simulink library "sm_scissor_lift_lib"  (R2020a)
settings: Solver=ode45  StartTime=0.0  StopTime=10.0  RelTol=1e-3  EnableMultiTasking=on
undefined symbols (not defined in the file): Extr_Data_Ring, Local, SCL_Par, X, Y, Z
libraries: sm_lib x38, $bdroot x37
(part 1 of 2)
Description:
  | Copyright 2014-2020 The MathWorks, Inc.
settings Model: Creator=smiller  LastModifiedBy=Vulca
settings DataIOCC: LimitDataPoints=on  SaveFormat=Array  SignalLoggingSaveFormat=ModelDataLogs  ReturnWorkspaceOutputs=off
settings OptimizationCC: ExpressionDepthLimit=2147483647  LifeSpan=inf
settings DebuggingCC: UnderspecifiedInitializationDetection=Classic  MergeDetectMultiDrivingBlocksExec=none  SolverPrmCheckMsg=warning  FcnCallInpInsideContextMsg=warning  AllowSymbolicDim=off  StateNameClashWarn=warning  PregeneratedLibrarySubsystemCodeDiagnostic=none  SFUnexpectedBacktrackingDiag=warning  SFNoUnconditionalDefaultTransitionDiag=warning  SFExecutionAtInitializationDiag=none  ArithmeticOperatorsInVariantConditions=warning
settings HardwareCC: ProdBitPerPointer=32  ProdBitPerSizeT=32  ProdBitPerPtrDiffT=32  ProdLargestAtomicFloat=None  ProdIntDivRoundTo=Undefined  ProdEndianess=Unspecified  ProdWordSize=32  ProdHWDeviceType=32-bit Generic
settings ModelReferenceCC: PropagateSignalLabelsOutOfModel=off
settings SFSimCC: SimUseLocalCustomCode=off  CustomCodeUndefinedFunction=UseInterfaceOnly
settings RTWCC: RTWUseLocalCustomCode=off
settings CodeAppCC: StateflowObjectComments=on
settings GRTTargetCC: TargetLangStandard=C89/C90 (ANSI)
settings ConfigComp: CovMetricSettings=dw  CovHtmlReporting=on  CovSaveCumulativeToWorkspaceVar=on  CovSaveSingleToWorkspaceVar=on  CovExternalEMLEnable=off  CovSFcnEnable=off

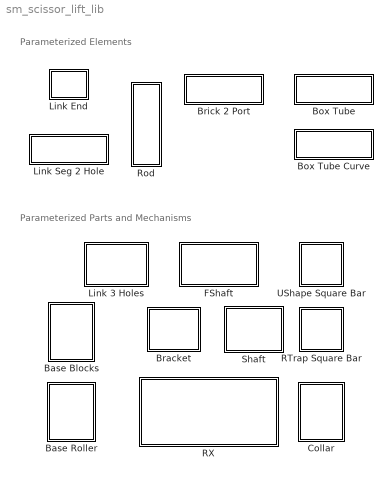
== system sm_scissor_lift_lib ==
  note: Parameterized Elements
  note: Parameterized Parts and Mechanisms
  Base Blocks : Subsystem  mask(Base Blocks){block_length=SCL_Par.Base_Block.Length, block_width=SCL_Par.Base_Block.Width, block_height=SCL_Par.Base_Block.Height, shaft_radius=SCL_Par.Roller.Shaft_Radius, shaft_length=SCL_Par.Roller.Shaft_Length, material_density=SCL_Par.Base_Block.Density, material_color=SCL_Par.Base_Block.Color, material_opacity=SCL_Par.Base_Block.Opacity}
      mask prompts: block_length "Length (cm)"; block_width "Width (cm)"; block_height "Height (cm)"; shaft_radius "Radius (cm)"; shaft_length "Length (cm)"; material_density "Density (kg/m^3)"; material_color "Color [RGB]"; material_opacity "Opacity (0-1)"
      mask help: Parameterized base with two blocks and a shaft.
      mask DialogControl ParameterTabVar0 Prompt: Block
      mask DialogControl ParameterTabVar01 Prompt: Shaft
      mask DialogControl ParameterTabVar012 Prompt: Material
      mask Display: image('Base_Blocks_IMAGE.jpg');
  Base Roller : Subsystem  mask(Base Roller){roller_length=SCL_Par.Roller.Roller_Length, roller_radius=SCL_Par.Roller.Roller_Radius, shaft_length=SCL_Par.Roller.Shaft_Length, shaft_radius=SCL_Par.Roller.Shaft_Radius, material_density=SCL_Par.Roller.Density, material_color=SCL_Par.Roller.Color, material_opacity=SCL_Par.Roller.Opacity}
      mask prompts: roller_length "Length (cm)"; roller_radius "Radius (cm)"; shaft_length "Length (cm)"; shaft_radius "Radius (cm)"; material_density "Density (kg/m^3)"; material_color "Color [RGB]"; material_opacity "Opacity (0-1)"
      mask help: Parameterized roller with two wheels connected by a shaft.
      mask DialogControl ParameterTabVar0 Prompt: Roller
      mask DialogControl ParameterTabVar01 Prompt: Shaft
      mask DialogControl ParameterTabVar012 Prompt: Material
      mask Display: image('Base_Roller_IMAGE.jpg');
  Box Tube : Subsystem  mask(Box Tube){box_ox=0.02, box_ix=0.01, box_oy=0.028, box_iy=0.018, box_len=0.5, box_rho=7000, box_color=[0 0.4 0.6], box_opc=1}
      mask prompts: box_len "Length (m)"; box_rho "Density (kg/m^3)"; box_color "Color [RGB]"; box_opc "Opacity (0-1)"
      mask help: Box tube. Define outer dimensions, inner dimensions, and length. Length defines the distance of the +X frame from the X frame along the x-axis.
      mask init:
      | box_xsec = Extr_Data_Box(box_ox, box_ix, box_oy, box_iy);
      mask DialogControl Control12 Prompt: Plot Profile
      mask DialogControl Control12 Callback:
      | v = get_param(gcb,'MaskWSVariables');
      | getMaskValue = containers.Map({v.Name}',{v.Value}');
      | evalin('base',...
      |     sprintf('Extr_Data_Box(%s,%s,%s,%s,''%s'');',...
      |     num2str(getMaskValue('box_ox')),...
      |     num2str(getMaskValue('box_ix')),...
      |     num2str(getMaskValue('box_oy')),...
      |     num2str(getMaskValue('box_iy')),'plot'));
      mask DialogControl Control3 Prompt: Outer
      mask DialogControl Control4 Prompt: Inner
      mask DialogControl Control5 Prompt: Width (m)
      mask DialogControl Control6 Prompt: Height (m)
      mask Display: image('Box_Tube_IMAGE.png');
  Box Tube Curve : Subsystem  mask(Box Tube with Curve){box_ox=0.02, box_ix=0.01, box_oy=0.028, box_iy=0.018, arc_rad=0.5, arc_angle=-60, popup_arcdir=Y, box_rho=7000, box_color=[0 0.4 0.6], box_opc=1}
      mask prompts: arc_rad "Arc Radius (m)"; arc_angle "Arc Angle (deg)"; popup_arcdir "About"; box_rho "Density (kg/m^3)"; box_color "Color [RGB]"; box_opc "Opacity (0-1)"
      mask help: Box tube. Define outer dimensions, inner dimensions, and length. Length defines the distance of the F frame from the B frame along the z-axis.
      mask init:
      | box_xsec = Extr_Data_Box(box_ox, box_ix, box_oy, box_iy);
      | 
      | % Transform extrusion data based on curve axis and direction
      | if (arc_angle<0)
      |     if(strcmpi(get_param(gcb,'popup_arcdir'),'y'))
      |         box_xsec_d = flipud(box_xsec.*[1 -1]);
      |         Bzrot = -90-arc_angle/2;
      |         Fzrot = -90+arc_angle/2;
      |     elseif(strcmpi(get_param(gcb,'popup_arcdir'),'z'))
      |         box_xsec_d = fliplr(box_xsec).*[1 -1];
      |         Bzrot = 90+arc_angle/2;
      |         Fzrot = -90+arc_angle/2;
      |     end
      | else
      |     if(strcmpi(get_param(gcb,'popup_arcdir'),'y'))
      |         box_xsec_d = flipud(box_xsec.*[-1 1]);
      |     elseif(strcmpi(get_param(gcb,'popup_arcdir'),'z'))
      |         box_xsec_d = -flipud(fliplr(box_xsec));
      |     end
      |     Bzrot = -90+arc_angle/2;
      |     Fzrot = 90+arc_angle/2;
      | end
      | 
      | % Add offset for arc radius
      | box_xsec_d = box_xsec_d + [arc_rad 0];
      | 
      | % Adjust Base and Follower transforms based on curve axis
      | if(strcmpi(get_param(gcb,'popup_arcdir'),'y'))
      |     set_param([gcb '/Transform B'],'TranslationStandardAxis','-Z');
      |     set_param([gcb '/Transform B'],'RotationSequenceAngles','[-90*sign(arc_angle) Bzrot 0]');
      |     set_param([gcb '/Transform F'],'RotationSequenceAngles','[90*sign(arc_angle) Fzrot 0]');
      |     set_param([gcb '/Transform F'],'TranslationThetaOffset','arc_angle/2*sign(arc_angle)')
      | else
      |     set_param([gcb '/Transform B'],'TranslationStandardAxis','+Y');
      |     set_param([gcb '/Transform B'],'RotationSequenceAngles','[0 Bzrot 0]');
      |     set_param([gcb '/Transform F'],'RotationSequenceAngles','[0 0 Fzrot]');
      |     set_param([gcb '/Transform F'],'TranslationThetaOffset','arc_angle/2');
      | end
      mask TypeOptions popup_arcdir: Y | Z
      mask DialogControl Control12 Prompt: Plot Profile
      mask DialogControl Control12 Callback:
      | v = get_param(gcb,'MaskWSVariables');
      | getMaskValue = containers.Map({v.Name}',{v.Value}');
      | evalin('base',...
      |     sprintf('Extr_Data_Box(%s,%s,%s,%s,''%s'');',...
      |     num2str(getMaskValue('box_ox')),...
      |     num2str(getMaskValue('box_ix')),...
      |     num2str(getMaskValue('box_oy')),...
      |     num2str(getMaskValue('box_iy')),'plot'));
      mask DialogControl Control3 Prompt: Outer
      mask DialogControl Control4 Prompt: Inner
      mask DialogControl Control5 Prompt: Width (m)
      mask DialogControl Control6 Prompt: Height (m)
      mask Display: image('Box_Tube_Curve_IMAGE.png')
  Bracket : Subsystem  mask(Actuation Bracket){fl_w=70, fl_h=13.5, T=4, w_link=15, offset_l=35, offset_h=15, flupdown=Down, flfrontrear=Rear, fl_density=1000, fl_clr=[0.9  0.9  0.9], fl_opc=1, shaft_length=60, shaft_radius=5, shaft_density=1000, shaft_color=[0.6431    0.7216    0.7843], shaft_opacity=1}
      mask prompts: fl_w "Width (cm)"; fl_h "Height (cm)"; T "Thickness (cm)"; w_link "Link Width (cm)"; offset_l "Offset Along Link (cm)"; offset_h "Offset from Link Centerline (cm)"; flupdown "Orientation"; flfrontrear "Position"; fl_density "Density (kg/m^3)"; fl_clr "Color [RGB]"; fl_opc "Opacity (0-1)"; shaft_length "Length (cm)"; shaft_radius "Radius (cm)"; shaft_density "Density (kg/m^3)"; shaft_color "Color [RGB]"; shaft_opacity "Opacity (0-1)"
      mask help: Actuation bracket for scissor lift mechanism. Contains flanges that attach to links and connection shaft. Configurable orientation and surface attachment.
      mask init:
      | if(flupdown == 2)
      |     flupdown = -1;
      | end
      | if(flfrontrear == 2)
      |     flfrontrear = -1;
      | end
      | 
      | flange_xsec = [...
      |     -shaft_radius-1 shaft_radius+1;...
      |     -fl_w/2           -(offset_h-w_link/2);...
      |      fl_w/2           -(offset_h-w_link/2);...
      |      shaft_radius+1 shaft_radius+1]*flupdown;
      |  
      | %    [0 fl_h+W; 
      | %    -fl_w -fl_h+W; 
      | %    fl_w -fl_h+W]*0.5*flupdown
      | %    
      | %    fl_h+W; -fl_w -fl_h+W; fl_w -fl_h+W]*0.5*flupdown
      mask TypeOptions flupdown: Down | Up
      mask TypeOptions flfrontrear: Front | Rear
      mask DialogControl ParameterTabVar0 Prompt: Flange Dims.
      mask DialogControl ParameterTabVar01 Prompt: Flange Matl.
      mask DialogControl ParameterTabVar012 Prompt: Shaft
      mask Display: image('Bracket_IMAGE.jpg');
  Brick 2 Port : Subsystem  mask(Brick with 2 Interface Frames){len_xyz=[0.1 0.2 0.3], brick_rho=7000, brick_clr=[0.6 0.6 0.6], brick_opc=1, popup_port1=+X, popup_port2=+X, port1_offset=[0 0 0]}
      mask prompts: len_xyz "Length [X Y Z] (m)"; brick_rho "Density (kg/m^3)"; brick_clr "Color [RGB]"; brick_opc "Opacity (0-1)"; popup_port1 "Port 1 Face"; popup_port2 "Port 2 Face"
      mask help: This block models a brick. The two interface ports can be configured to be at the center of any of the six faces. The orientation of the frames is the same.
      mask init:
      | p1_h = char(find_system(gcb,'FollowLinks','on','LookUnderMasks','all','Port','1'));
      | p2_h = char(find_system(gcb,'FollowLinks','on','LookUnderMasks','all','Port','2'));
      | switch(popup_port1)
      |     case 1, port1_offset = [ len_xyz(1)/2 0 0]; port1_name = '1X';
      |     case 2, port1_offset = [-len_xyz(1)/2 0 0];  port1_name = '1-X';
      |     case 3, port1_offset = [ 0  len_xyz(2)/2 0];  port1_name = '1Y';
      |     case 4, port1_offset = [ 0 -len_xyz(2)/2 0];  port1_name = '1-Y';
      |     case 5, port1_offset = [ 0  0  len_xyz(3)/2]; port1_name = '1Z';
      |     case 6, port1_offset = [ 0  0 -len_xyz(3)/2]; port1_name = '1-Z';
      | end
      | 
      | switch(popup_port2)
      |     case 1, port2_offset = [ len_xyz(1)/2 0 0]; port2_name = 'X2';
      |     case 2, port2_offset = [-len_xyz(1)/2 0 0];  port2_name = '-X2';
      |     case 3, port2_offset = [ 0  len_xyz(2)/2 0];  port2_name = 'Y2';
      |     case 4, port2_offset = [ 0 -len_xyz(2)/2 0];  port2_name = '-Y2';
      |     case 5, port2_offset = [ 0  0  len_xyz(3)/2]; port2_name = 'Z2';
      |     case 6, port2_offset = [ 0  0 -len_xyz(3)/2]; port2_name = '-Z2';
      | end
      | 
      | set_param(p1_h,'Name',port1_name);
      | set_param(p2_h,'Name',port2_name);
      mask TypeOptions popup_port1: +X | -X | +Y | -Y | +Z | -Z
      mask TypeOptions popup_port2: +X | -X | +Y | -Y | +Z | -Z
      mask Display: image('Brick_2_Port_IMAGE.png')
  Collar : Subsystem  mask{collar_length=30, collar_radius=5.5, cylinder_length=129.6, cylinder_radius=5.5, cylinder_ori=Local +Z, material_density=1000, material_color=[0.5 0.5 0.5], material_opacity=1}
      mask prompts: collar_length "Length (cm):"; collar_radius "Radius (cm):"; cylinder_length "Length (cm):"; cylinder_radius "Radius (cm):"; cylinder_ori "Orientation (B to C):"; material_density "Density (kg/m^3):"; material_color "Color:"; material_opacity "Opacity:"
      mask init:
      | if(cylinder_ori == 2)
      |     cylinder_ori = -1;
      | end
      mask TypeOptions cylinder_ori: Local +Z | Local -Z
      mask DialogControl ParameterTabVar0 Prompt: Collar
      mask DialogControl ParameterTabVar01 Prompt: Cylinder
      mask DialogControl ParameterTabVar012 Prompt: Material
      mask Display: image('Actuator_Collar_IMAGE.jpg');
  FShaft : Subsystem  mask(Transverse Shaft){sep_outer_outer=80, sep_outer_inner=10, shaft_radius=5, shaft_density=1000, shaft_color=[0.6431    0.7216    0.7843], shaft_opacity=1}
      mask prompts: sep_outer_outer "Outer connection separation (cm)"; sep_outer_inner "Outer to inner separation (cm)"; shaft_radius "Radius (cm)"; shaft_density "Density (kg/m^3)"; shaft_color "Color [R G B]"; shaft_opacity "Opacity (0-1)"
      mask help: Transverse shaft with four connections. Frames are located at shaft center, with Z-axis along center.
      mask DialogControl ParameterTabVar0 Prompt: Connections
      mask DialogControl ParameterTabVar01 Prompt: Shaft
      mask Display: image('Shaft_IMAGE.jpg');
  Link 3 Holes : Subsystem  mask(Connector Link, 3 Holes){L=240, W=15, T=4, r=5, rho=1000, clr_string=Gray, opc=1}
      mask prompts: L "Link length (cm):"; W "Link width (cm):"; T "Link thickness (cm):"; r "Hole radius (cm):"; rho "Density (kg/m^3):"; clr_string "Color:"; opc "Opacity:"
      mask help: Connector link with holes. Ports are located at centers of holes, oriented such that Z is out of the hole, positive X is from L hole to R hole.
      mask init:
      | imgfile='Link_3_Hole_Yellow_IMAGE.jpg';
      | if(strcmp(clr_string,'Yellow'))
      |     clr = [0.6 0.6 0.0];
      | elseif(strcmp(clr_string,'Red'))
      |     clr = [0.8 0.2 0.0];
      |     imgfile='Link_3_Hole_Red_IMAGE.jpg';
      | elseif(strcmp(clr_string,'Gray'))
      |     clr = [0.9 0.9 0.9];
      |     imgfile='Link_3_Hole_Gray_IMAGE.jpg';
      | elseif(strcmp(clr_string,'Gray-Blue'))
      |     clr = [164 184 200]/255;
      |     imgfile='Link_3_Hole_GrayBlue_IMAGE.jpg';
      | end
      mask TypeOptions clr_string: Yellow | Red | Gray | Gray-Blue
      mask DialogControl ParameterTabVar0 Prompt: Dimensions
      mask DialogControl ParameterTabVar01 Prompt: Material
      mask Display: image(imread(imgfile));
  Link End : Subsystem  mask(Link End){circ_radout=0.025/2, circ_radin=0.005, popup_holelr=-X, deg_1=90, deg_2=270, circ_len=0.01, circ_rho=7000, circ_color=[0 0.4 0.6], circ_opc=1}
      mask prompts: circ_radout "Outer Radius (m)"; circ_radin "Hole Radius (m)"; popup_holelr "Hole Side"; deg_1 "Start Angle (deg)"; deg_2 "Finish Angle (deg)"; circ_len "Thickness (m)"; circ_rho "Density (kg/m^3)"; circ_color "Color [RGB]"; circ_opc "Opacity (0-1)"
      mask help: Round end of Link. Define outer radius, hole radius, and hole placement. Port is at the hole center.
      mask init:
      | port_h=find_system(gcb,'regexp','on','FollowLinks','on',...
      |     'LookUnderMasks','on','Side','.*');
      | if(strcmpi(get_param(gcb,'popup_holelr'),'+X'));
      |     set_param(gcb,'deg_1','-90','deg_2','90');
      |     set_param(char(port_h),'Name','+X');
      | else
      |     set_param(gcb,'deg_1','90','deg_2','270');
      |     set_param(char(port_h),'Name','X');
      | end
      | circ_xsec = Extr_Data_Ring(circ_radout, circ_radin, deg_1, deg_2);
      mask TypeOptions popup_holelr: -X | +X
      mask DialogControl Control12 Prompt: Plot Profile
      mask DialogControl Control12 Callback:
      | v = get_param(gcb,'MaskWSVariables');
      | getMaskValue = containers.Map({v.Name}',{v.Value}');
      | 
      | if(strcmp(get_param(gcb,'popup_holelr'),'+X'))
      |     evalin('base',...
      |         sprintf('Extr_Data_Ring(%s,%s,%s,%s,''%s'');',...
      |         num2str(getMaskValue('circ_radout')),...
      |         num2str(getMaskValue('circ_radin')),...
      |         '-90',...
      |         '90','plot'));
      | else
      |     evalin('base',...
      |         sprintf('Extr_Data_Ring(%s,%s,%s,%s,''%s'');',...
      |         num2str(getMaskValue('circ_radout')),...
      |         num2str(getMaskValue('circ_radin')),...
      |         '90',...
      |         '270','plot'));
      | end
      mask Display:
      | if(strcmp(get_param(gcb,'popup_holelr'),'+X'))
      |     image('Link_End_px_IMAGE.png');
      | else
      |     image('Link_End_nx_IMAGE.png');
      | end
  Link Seg 2 Hole : Subsystem  mask(Link Segment with 2 Holes){link_len=0.05, link_width=0.025, link_radh=0.005, link_thickness=0.01, link_rho=7000, link_color=[0 0.4 0.6], link_opc=1}
      mask prompts: link_len "Length (m)"; link_width "Width (m)"; link_radh "Hole Radius (m)"; link_thickness "Thickness (m)"; link_rho "Density (kg/m^3)"; link_color "Color [RGB]"; link_opc "Opacity (0-1)"
      mask help: Link segment with one hole. Define outer dimensions and hole radius. The interface ports are at either end of the link segment.
      mask init:
      | link_xsec = Extr_Data_Link2Hole(link_len, link_width, link_radh);
      mask DialogControl Control12 Prompt: Plot Profile
      mask DialogControl Control12 Callback:
      | v = get_param(gcb,'MaskWSVariables');
      | getMaskValue = containers.Map({v.Name}',{v.Value}');
      | evalin('base',...
      |     sprintf('Extr_Data_Link2Hole(%s,%s,%s,''%s'');',...
      |     num2str(getMaskValue('link_len')),...
      |     num2str(getMaskValue('link_width')),...
      |     num2str(getMaskValue('link_radh')),'plot'));
      mask Display: image('Link_Seg_2_Hole_IMAGE.png');
  RTrap Square Bar : Subsystem  mask(U-Shape from Round Bar){pipe_width=5, height_c1=30, height_c2=60, rail_curve_rad1=20, rail_curve_rad2=20, curve_ang1=60, curve_ang2=45, width=150, clr=[0 0.6 0.8], rho=0.01}
      mask prompts: pipe_width "Pipe Width (cm)"; width "Width (cm)"; clr "Color"; rho "Density"
      mask help: U-Shape formed from a bar with square cross-section
      mask DialogControl Container7 Prompt: Dimensions
      mask DialogControl Control2 Prompt: Curve 1
      mask DialogControl Control3 Prompt: Curve 2
      mask DialogControl Control7 Prompt: Height (cm)
      mask DialogControl Control8 Prompt: Curve Radius (cm)
      mask DialogControl Control9 Prompt: Angle (deg)
      mask DialogControl Container5 Prompt: Material
      mask Display: image('Trap_Shaped_Rail_IMAGE.png')
  RX : Subsystem  mask(Scissor Lift Crossbar){leftright=Right, link_length_in=240, link_length_out=240, link_width_in=15, link_width_out=15, link_thickness_in=4, link_thickness_out=4, link_hole_radius_in=5, link_hole_radius_out=5, link_density_in=10, link_density_out=10, link_color_in=[0.9 0.9 0.9], link_color_out=[0.6431 0.7216  0.7843], link_opacity_in=1, link_opacity_out=1, shaft_length=10, shaft_radius=5, shaft_density=1000, shaft_color=[0.6431 0.7216 0.7843], shaft_opacity=1, imgfile=Crossbar_RX_IMAGE.jpg}
      mask prompts: leftright "Side"; shaft_length "Length (cm)"; shaft_radius "Radius (cm)"; shaft_density "Density (kg/m^3)"; shaft_color "Color"; shaft_opacity "Opacity"; imgfile "Image File"
      mask help: Parameterized crossbar. The two links are connected by a revolute joint. Configurable for left or right side.
      mask init:
      | pinbpth = [gcb '/Pin'];
      | if (leftright == 1)
      |     set_param(char(pinbpth),'popup_zori','Local -Z');
      |     set_param([gcb '/OL'],'Port','2','Side','Right');
      |     set_param([gcb '/IL'],'Port','1','Side','Right');
      |     set_param([gcb '/OU'],'Port','4','Side','Left');
      |     set_param([gcb '/IU'],'Port','3','Side','Left');
      |     set_param(gcb,'Name','RX');
      |     imgfile = 'Crossbar_LX_IMAGE.jpg';
      | else
      |     set_param(char(pinbpth),'popup_zori','Local +Z');
      |     set_param([gcb '/IL'],'Port','2','Side','Right');
      |     set_param([gcb '/OL'],'Port','1','Side','Right');
      |     set_param([gcb '/IU'],'Port','4','Side','Left');
      |     set_param([gcb '/OU'],'Port','3','Side','Left');
      |     set_param(gcb,'Name','LX');
      |     imgfile = 'Crossbar_RX_IMAGE.jpg';
      | end
      mask TypeOptions leftright: Right | Left
      mask DialogControl ParameterTabVar0 Prompt: Links
      mask DialogControl text_Inner Prompt: Inner
      mask DialogControl text_Outer Prompt: Outer
      mask DialogControl text_Length Prompt: Length (cm)
      mask DialogControl text_Width Prompt: Width (cm)
      mask DialogControl text_Thickness Prompt: Thickness (cm)
      mask DialogControl text_hole_radius Prompt: Hole Radius (cm)
      mask DialogControl text_density Prompt: Density (kg/m^3)
      mask DialogControl text_color Prompt: Color [RGB]
      mask DialogControl text_opacity Prompt: Opacity (0-1)
      mask DialogControl ParameterTabVar01 Prompt: Shaft
      mask Display: image(imgfile);
  Rod : Subsystem  mask(Rod){rod_rad=0.005, rod_len=0.0125, rod_rho=7000, rod_color=[0.5 0.5 0.5], rod_opc=1, popup_zori=Local +Z, popup_markings=None, mark_radius_range=[0.5 1.01], mark_length_range=1.005, mark_angle_range=30, mark_color=[1 1 1]}
      mask prompts: rod_rad "Radius (m)"; rod_len "Length (m)"; rod_rho "Density (kg/m^3)"; rod_color "Color [RGB]"; rod_opc "Opacity (0-1)"; popup_zori "Relative Position (B to F)"; popup_markings "Show Markings"; mark_radius_range "Radial Range [min max] (0-1.1)"; mark_length_range "Length Range (0-1.1)"; mark_angle_range "Sweep Angle [0-180] (deg)"; mark_color "Color [RGB]"
      mask help:
      | This block models a rod.
      |
      | The two interface ports corresponds to the frames at either end of the rod which are along the z-axis.
      mask init:
      | mark_xsec =  [
      |     rod_rad*max(mark_radius_range) rod_len*mark_length_range/2; 
      |     rod_rad*min(mark_radius_range) rod_len*mark_length_range/2; 
      |     rod_rad*min(mark_radius_range) -rod_len*mark_length_range/2; 
      |     rod_rad*max(mark_radius_range) -rod_len*mark_length_range/2];
      | 
      | mark_1_opc = 0;
      | mark_2_opc = 0;
      | 
      | if(popup_markings == 2)
      |     mark_1_opc = 1;
      | elseif(popup_markings == 3)
      |     mark_1_opc = 1;
      |     mark_2_opc = 1;
      | end
      | 
      | if(popup_zori == 2)
      |     z_ori = -1;
      | else
      |     z_ori = 1;
      | end
      mask TypeOptions popup_zori: Local +Z | Local -Z
      mask TypeOptions popup_markings: None | One | Two
      mask Callback popup_markings:
      | maskObj = Simulink.Mask.get(gcb);
      | mkc_h = maskObj.getDialogControl('container_markings');
      | if strcmp(get_param(gcb,'popup_markings'),'None')
      |     mkc_h.Visible = 'off';
      | else
      |     mkc_h.Visible = 'on';
      | end
      | clear maskObj mkc_h
      mask Display:
      | if(popup_zori == 2)
      |     image('Rod_nZ_IMAGE.png')
      | else
      |     image('Rod_pZ_IMAGE.png')
      | end
  Shaft : Subsystem  mask(Cylindrical Shaft){L=10, r=5, theta=0, z_ori=Local -Z, Ro=1000, clr=[0.6431    0.7216    0.7843], opc=1}
      mask prompts: L "Length (cm):"; r "Radius (cm):"; theta "Twist (deg)"; z_ori "Orientation (B to F)"; Ro "Density (kg/m^3):"; clr "Color:"; opc "Opacity"
      mask help: Cylindrical shaft. Ports are at shaft ends, and oriented such that the Z-axis is between the ports. Can be configured to have positive Z from B to F or from F to B.
      mask init:
      | if(z_ori == 2)
      |     z_ori = -1;
      | end
      mask TypeOptions z_ori: Local +Z | Local -Z
      mask DialogControl ParameterTabVar0 Prompt: Dimensions
      mask DialogControl ParameterTabVar01 Prompt: Material
      mask Display: image('Shaft_IMAGE.jpg');
  UShape Square Bar : Subsystem  mask(U-Shape from Round Bar){pipe_width=2.5, rail_curve_rad=20, height=150, width=280, clr=[0 0.6 0.8], rho=0.01}
      mask prompts: pipe_width "Pipe Width (cm)"; rail_curve_rad "Rail Curve Radius (cm)"; height "Height (cm)"; width "Width (cm)"; clr "Color"; rho "Density"
      mask help: U-Shape formed from a bar with square cross-section
      mask DialogControl Container7 Prompt: Dimensions
      mask DialogControl Container5 Prompt: Material
      mask Display: image('U_Shaped_Rail_IMAGE.png')

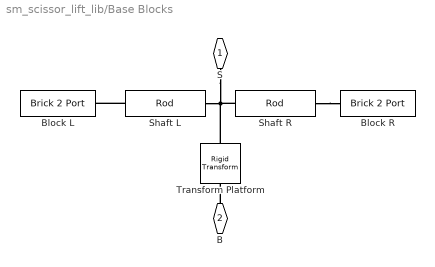
== system sm_scissor_lift_lib/Base Blocks ==
  Block L : $bdroot/Brick 2 Port  len_xyz=[block_width block_height block_length]*1e-2  brick_rho=material_density  brick_clr=material_color  brick_opc=1  popup_port1=-Z  popup_port2=+Z  port1_offset=[0 0 0]
  Block R : $bdroot/Brick 2 Port  len_xyz=[block_width block_height block_length]*1e-2  brick_rho=material_density  brick_clr=material_color  brick_opc=1  popup_port1=+Z  popup_port2=-Z  port1_offset=[0 0 0]
  Shaft L : $bdroot/Rod  rod_rad=shaft_radius*1e-2  rod_len=shaft_length/2*1e-2  rod_rho=material_density  rod_color=material_color  rod_opc=material_opacity  popup_zori=Local -Z  popup_markings=None  mark_radius_range=[0.5 1.01]  mark_length_range=1.005  mark_angle_range=30  mark_color=[1 1 1]
  Shaft R : $bdroot/Rod  rod_rad=shaft_radius*1e-2  rod_len=shaft_length/2*1e-2  rod_rho=material_density  rod_color=material_color  rod_opc=material_opacity  popup_zori=Local +Z  popup_markings=None  mark_radius_range=[0.5 1.01]  mark_length_range=1.005  mark_angle_range=30  mark_color=[1 1 1]
  Transform Platform : sm_lib/Frames and Transforms/Rigid Transform  TranslationMethod=Cartesian  TranslationStandardOffset=1  TranslationLengthUnit=cm  TranslationStandardAxis=-Y  TranslationCartesianOffset=[0 -block_height/2 0]  TranslationROffset=0  TranslationROffsetUnits=m  TranslationZOffset=0  TranslationZOffsetUnits=m  TranslationThetaOffset=0  TranslationThetaOffsetUnits=deg  RotationMethod=None  RotationAngleUnits=deg  RotationStandardAxis=+Y  RotationAngle=0  RotationArbitraryAxis=[0 0 1]  FollAlignAxisA=+X  BaseAlignAxisA=+Y  FollAlignAxisB=+Y  BaseAlignAxisB=+Z  RotationSequenceAxes=FollowerAxes  RotationSequence=XYX  RotationSequenceAngles=[0 0 0]  RotationSequenceAnglesUnits=deg  RotationMatrix=[1 0 0; 0 1 0; 0 0 1]
  S : PMIOPort  Side=Right
  B : PMIOPort  Port=2  Side=Left
  connections:
  S/RConn1 -- Shaft R/LConn1 -- Shaft L/LConn1 -- Transform Platform/LConn1
  B/RConn1 -- Transform Platform/RConn1
  Shaft R/RConn1 -- Block R/RConn1
  Shaft L/RConn1 -- Block L/RConn1

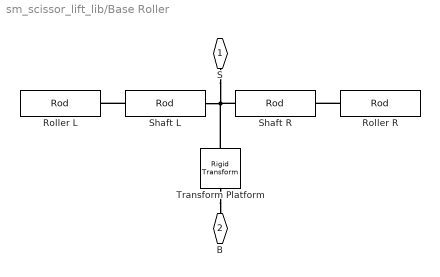
== system sm_scissor_lift_lib/Base Roller ==
  Roller L : $bdroot/Rod  rod_rad=roller_radius*1e-2  rod_len=roller_length*1e-2  rod_rho=material_density  rod_color=material_color  rod_opc=material_opacity  popup_zori=Local -Z  popup_markings=None  mark_radius_range=[0.5 1.01]  mark_length_range=1.005  mark_angle_range=30  mark_color=[1 1 1]
  Roller R : $bdroot/Rod  rod_rad=roller_radius*1e-2  rod_len=roller_length*1e-2  rod_rho=material_density  rod_color=material_color  rod_opc=material_opacity  popup_zori=Local +Z  popup_markings=None  mark_radius_range=[0.5 1.01]  mark_length_range=1.005  mark_angle_range=30  mark_color=[1 1 1]
  Shaft L : $bdroot/Rod  rod_rad=shaft_radius*1e-2  rod_len=shaft_length/2*1e-2  rod_rho=material_density  rod_color=material_color  rod_opc=material_opacity  popup_zori=Local -Z  popup_markings=None  mark_radius_range=[0.5 1.01]  mark_length_range=1.005  mark_angle_range=30  mark_color=[1 1 1]
  Shaft R : $bdroot/Rod  rod_rad=shaft_radius*1e-2  rod_len=shaft_length/2*1e-2  rod_rho=material_density  rod_color=material_color  rod_opc=material_opacity  popup_zori=Local +Z  popup_markings=None  mark_radius_range=[0.5 1.01]  mark_length_range=1.005  mark_angle_range=30  mark_color=[1 1 1]
  Transform Platform : sm_lib/Frames and Transforms/Rigid Transform  TranslationMethod=None  TranslationStandardOffset=0  TranslationLengthUnit=cm  TranslationStandardAxis=-Y  TranslationCartesianOffset=[0 0 0]  TranslationROffset=0  TranslationROffsetUnits=m  TranslationZOffset=0  TranslationZOffsetUnits=m  TranslationThetaOffset=0  TranslationThetaOffsetUnits=deg  RotationMethod=StandardAxis  RotationAngleUnits=deg  RotationStandardAxis=+Y  RotationAngle=90  RotationArbitraryAxis=[0 0 1]  FollAlignAxisA=+X  BaseAlignAxisA=+Y  FollAlignAxisB=+Y  BaseAlignAxisB=+Z  RotationSequenceAxes=FollowerAxes  RotationSequence=XYX  RotationSequenceAngles=[0 0 0]  RotationSequenceAnglesUnits=deg  RotationMatrix=[1 0 0; 0 1 0; 0 0 1]
  S : PMIOPort  Side=Right
  B : PMIOPort  Port=2  Side=Left
  connections:
  Transform Platform/RConn1 -- B/RConn1
  Transform Platform/LConn1 -- Shaft R/LConn1 -- Shaft L/LConn1 -- S/RConn1
  Roller R/LConn1 -- Shaft R/RConn1
  Shaft L/RConn1 -- Roller L/LConn1

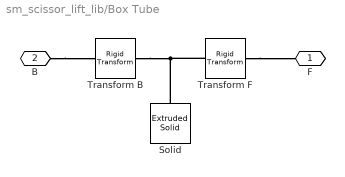
== system sm_scissor_lift_lib/Box Tube ==
  Solid : sm_lib/Body Elements/Extruded Solid  GraphicAmbientColor=[0.15 0.15 0.15 1.0]  BasedOnType=Density  CenterOfMass=[0 0 0]  CenterOfMassUnits=m  GraphicDiffuseColor=box_color  ExportConvexHullGeometry=off  ExtrusionCrossSection=box_xsec  ExtrusionCrossSectionUnits=m  Density=box_rho  DensityUnits=kg/(m^3)  DoExposeReferenceFrame=on  GraphicEmissiveColor=[0.0 0.0 0.0 1.0]  ExportEntireGeometry=off  ExtrusionLength=box_len  ExtrusionLengthUnits=m  ExtrusionType=General  SerializedFrames=<Frames/>  MarkerShape=Sphere  MarkerSize=10  GraphicType=FromGeometry  InertiaType=CalculateFromGeometry  Mass=1  MassUnits=kg  MomentsOfInertia=[1 1 1]  MomentsOfInertiaUnits=kg*m^2  PolygonNumSides=3  GraphicOpacity=box_opc  PolygonOuterRadius=1  PolygonOuterRadiusUnits=m  ProductsOfInertia=[0 0 0]  ProductsOfInertiaUnits=kg*m^2  GraphicShininess=75  GraphicSpecularColor=[0.5 0.5 0.5 1.0]  GraphicVisPropType=SimpleVisualProperties
  Transform B : sm_lib/Frames and Transforms/Rigid Transform  TranslationMethod=StandardAxis  TranslationStandardOffset=box_len/2  TranslationLengthUnit=m  TranslationStandardAxis=+X  TranslationCartesianOffset=[0 0 0]  TranslationROffset=0  TranslationROffsetUnits=m  TranslationZOffset=0  TranslationZOffsetUnits=m  TranslationThetaOffset=0  TranslationThetaOffsetUnits=deg  RotationMethod=StandardAxis  RotationAngleUnits=deg  RotationStandardAxis=+Y  RotationAngle=90  RotationArbitraryAxis=[0 0 1]  FollAlignAxisA=+X  BaseAlignAxisA=+Y  FollAlignAxisB=+Y  BaseAlignAxisB=+Z  RotationSequenceAxes=FollowerAxes  RotationSequence=XYX  RotationSequenceAngles=[0 0 0]  RotationSequenceAnglesUnits=deg  RotationMatrix=[1 0 0; 0 1 0; 0 0 1]
  Transform F : sm_lib/Frames and Transforms/Rigid Transform  TranslationMethod=StandardAxis  TranslationStandardOffset=box_len/2  TranslationLengthUnit=m  TranslationStandardAxis=+Z  TranslationCartesianOffset=[0 0 0]  TranslationROffset=0  TranslationROffsetUnits=m  TranslationZOffset=0  TranslationZOffsetUnits=m  TranslationThetaOffset=0  TranslationThetaOffsetUnits=deg  RotationMethod=StandardAxis  RotationAngleUnits=deg  RotationStandardAxis=+Y  RotationAngle=-90  RotationArbitraryAxis=[0 0 1]  FollAlignAxisA=+X  BaseAlignAxisA=+Y  FollAlignAxisB=+Y  BaseAlignAxisB=+Z  RotationSequenceAxes=FollowerAxes  RotationSequence=XYX  RotationSequenceAngles=[0 0 0]  RotationSequenceAnglesUnits=deg  RotationMatrix=[1 0 0; 0 1 0; 0 0 1]
  F : PMIOPort  Side=Right
  B : PMIOPort  Port=2  Side=Left
  connections:
  B/RConn1 -- Transform B/LConn1
  Transform F/RConn1 -- F/RConn1
  Transform B/RConn1 -- Solid/RConn1 -- Transform F/LConn1

== system sm_scissor_lift_lib/Box Tube Curve ==
  Solid : sm_lib/Body Elements/Revolved Solid  GraphicAmbientColor=[0.15 0.15 0.15 1.0]  BasedOnType=Density  CenterOfMass=[0 0 0]  CenterOfMassUnits=m  GraphicDiffuseColor=box_color  ExportConvexHullGeometry=off  Density=box_rho  DensityUnits=kg/m^3  DoExposeReferenceFrame=on  GraphicEmissiveColor=[0.0 0.0 0.0 1.0]  ExportEntireGeometry=off  SerializedFrames=<Frames/>  MarkerShape=Sphere  MarkerSize=10  GraphicType=FromGeometry  InertiaType=CalculateFromGeometry  Mass=1  MassUnits=kg  MomentsOfInertia=[1 1 1]  MomentsOfInertiaUnits=kg*m^2  GraphicOpacity=box_opc  ProductsOfInertia=[1 1 1]  ProductsOfInertiaUnits=kg*m^2  RevolutionCrossSection=box_xsec_d  RevolutionCrossSectionUnits=m  RevolutionAngle=abs(arc_angle)  RevolutionAngleUnits=deg  RevolutionExtent=Custom  GraphicShininess=75  GraphicSpecularColor=[0.5 0.5 0.5 1.0]  GraphicVisPropType=SimpleVisualProperties
  Transform B : sm_lib/Frames and Transforms/Rigid Transform  TranslationMethod=StandardAxis  TranslationStandardOffset=arc_rad*sign(arc_angle)  TranslationLengthUnit=m  TranslationStandardAxis=-Z  TranslationCartesianOffset=[-0.0155 0.074 0.1]  TranslationROffset=0  TranslationROffsetUnits=m  TranslationZOffset=0  TranslationZOffsetUnits=m  TranslationThetaOffset=0  TranslationThetaOffsetUnits=deg  RotationMethod=RotationSequence  RotationAngleUnits=deg  RotationStandardAxis=-X  RotationAngle=90  RotationArbitraryAxis=[0 0 1]  FollAlignAxisA=+Z  BaseAlignAxisA=+Y  FollAlignAxisB=+X  BaseAlignAxisB=+Z  RotationSequenceAxes=FollowerAxes  RotationSequence=XZX  RotationSequenceAngles=[-90*sign(arc_angle) Bzrot 0]  RotationSequenceAnglesUnits=deg  RotationMatrix=[1 0 0; 0 1 0; 0 0 1]
  Transform F : sm_lib/Frames and Transforms/Rigid Transform  TranslationMethod=Cylindrical  TranslationStandardOffset=0  TranslationLengthUnit=m  TranslationStandardAxis=+X  TranslationCartesianOffset=[-0.0155 0.074 0.1]  TranslationROffset=arc_rad  TranslationROffsetUnits=m  TranslationZOffset=0  TranslationZOffsetUnits=m  TranslationThetaOffset=arc_angle/2*sign(arc_angle)  TranslationThetaOffsetUnits=deg  RotationMethod=RotationSequence  RotationAngleUnits=deg  RotationStandardAxis=-X  RotationAngle=90  RotationArbitraryAxis=[0 0 1]  FollAlignAxisA=+Z  BaseAlignAxisA=+Y  FollAlignAxisB=+X  BaseAlignAxisB=+Z  RotationSequenceAxes=FollowerAxes  RotationSequence=XYZ  RotationSequenceAngles=[90*sign(arc_angle) Fzrot 0]  RotationSequenceAnglesUnits=deg  RotationMatrix=[1 0 0; 0 1 0; 0 0 1]
  F : PMIOPort  Side=Right
  B : PMIOPort  Port=2  Side=Left
  connections:
  Transform B/RConn1 -- Solid/RConn1 -- Transform F/LConn1
  Transform B/LConn1 -- B/RConn1
  Transform F/RConn1 -- F/RConn1

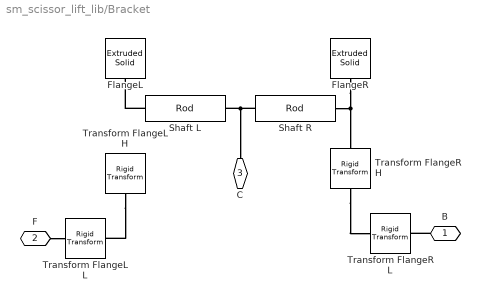
== system sm_scissor_lift_lib/Bracket ==
  FlangeL : sm_lib/Body Elements/Extruded Solid  GraphicAmbientColor=[0.5 0.5 0.5]  BasedOnType=Density  CenterOfMass=[0 0 0]  CenterOfMassUnits=m  GraphicDiffuseColor=fl_clr  ExportConvexHullGeometry=off  ExtrusionCrossSection=flange_xsec  ExtrusionCrossSectionUnits=cm  Density=fl_density  DensityUnits=kg/m^3  DoExposeReferenceFrame=on  GraphicEmissiveColor=[0.1 0.1 0.1]  ExportEntireGeometry=off  ExtrusionLength=T  ExtrusionLengthUnits=cm  ExtrusionType=General  SerializedFrames=<Frames/>  MarkerShape=Sphere  MarkerSize=1  GraphicType=FromGeometry  InertiaType=CalculateFromGeometry  Mass=1  MassUnits=kg  MomentsOfInertia=[1 1 1]  MomentsOfInertiaUnits=kg*m^2  PolygonNumSides=1  GraphicOpacity=fl_opc  PolygonOuterRadius=1  PolygonOuterRadiusUnits=m  ProductsOfInertia=[0 0 0]  ProductsOfInertiaUnits=kg*m^2  GraphicShininess=24.0  GraphicSpecularColor=[0.2 0.2 0.2]  GraphicVisPropType=SimpleVisualProperties
  FlangeR : sm_lib/Body Elements/Extruded Solid  GraphicAmbientColor=[0.5 0.5 0.5]  BasedOnType=Density  CenterOfMass=[0 0 0]  CenterOfMassUnits=m  GraphicDiffuseColor=fl_clr  ExportConvexHullGeometry=off  ExtrusionCrossSection=flange_xsec  ExtrusionCrossSectionUnits=cm  Density=fl_density  DensityUnits=kg/m^3  DoExposeReferenceFrame=on  GraphicEmissiveColor=[0.1 0.1 0.1]  ExportEntireGeometry=off  ExtrusionLength=T  ExtrusionLengthUnits=cm  ExtrusionType=General  SerializedFrames=<Frames/>  MarkerShape=Sphere  MarkerSize=1  GraphicType=FromGeometry  InertiaType=CalculateFromGeometry  Mass=1  MassUnits=kg  MomentsOfInertia=[1 1 1]  MomentsOfInertiaUnits=kg*m^2  PolygonNumSides=1  GraphicOpacity=fl_opc  PolygonOuterRadius=1  PolygonOuterRadiusUnits=m  ProductsOfInertia=[0 0 0]  ProductsOfInertiaUnits=kg*m^2  GraphicShininess=24.0  GraphicSpecularColor=[0.2 0.2 0.2]  GraphicVisPropType=SimpleVisualProperties
  Shaft L : $bdroot/Rod  rod_rad=shaft_radius*1e-2  rod_len=shaft_length/2*1e-2  rod_rho=shaft_density  rod_color=shaft_color  rod_opc=1  popup_zori=Local -Z  popup_markings=None  mark_radius_range=[0.5 1.01]  mark_length_range=1.005  mark_angle_range=30  mark_color=[1 1 1]
  Shaft R : $bdroot/Rod  rod_rad=shaft_radius*1e-2  rod_len=shaft_length/2*1e-2  rod_rho=shaft_density  rod_color=shaft_color  rod_opc=1  popup_zori=Local -Z  popup_markings=None  mark_radius_range=[0.5 1.01]  mark_length_range=1.005  mark_angle_range=30  mark_color=[1 1 1]
  Transform FlangeL H : sm_lib/Frames and Transforms/Rigid Transform  TranslationMethod=StandardAxis  TranslationStandardOffset=offset_h*flupdown  TranslationLengthUnit=cm  TranslationStandardAxis=+Y  TranslationCartesianOffset=[0 0 0]  TranslationROffset=0  TranslationROffsetUnits=m  TranslationZOffset=0  TranslationZOffsetUnits=m  TranslationThetaOffset=0  TranslationThetaOffsetUnits=deg  RotationMethod=None  RotationAngleUnits=deg  RotationStandardAxis=+Z  RotationAngle=0.0  RotationArbitraryAxis=[0 0 1]  FollAlignAxisA=+X  BaseAlignAxisA=+Y  FollAlignAxisB=+Y  BaseAlignAxisB=+Z  RotationSequenceAxes=FollowerAxes  RotationSequence=XYX  RotationSequenceAngles=[0 0 0]  RotationSequenceAnglesUnits=deg  RotationMatrix=[1 0 0; 0 1 0; 0 0 1]
  Transform FlangeL L : sm_lib/Frames and Transforms/Rigid Transform  TranslationMethod=StandardAxis  TranslationStandardOffset=(offset_l)*flfrontrear  TranslationLengthUnit=cm  TranslationStandardAxis=+X  TranslationCartesianOffset=[0 0 0]  TranslationROffset=0  TranslationROffsetUnits=m  TranslationZOffset=0  TranslationZOffsetUnits=m  TranslationThetaOffset=0  TranslationThetaOffsetUnits=deg  RotationMethod=None  RotationAngleUnits=deg  RotationStandardAxis=+Z  RotationAngle=0.0  RotationArbitraryAxis=[0 0 1]  FollAlignAxisA=+X  BaseAlignAxisA=+Y  FollAlignAxisB=+Y  BaseAlignAxisB=+Z  RotationSequenceAxes=FollowerAxes  RotationSequence=XYX  RotationSequenceAngles=[0 0 0]  RotationSequenceAnglesUnits=deg  RotationMatrix=[1 0 0; 0 1 0; 0 0 1]
  Transform FlangeR H : sm_lib/Frames and Transforms/Rigid Transform  TranslationMethod=StandardAxis  TranslationStandardOffset=offset_h*flupdown  TranslationLengthUnit=cm  TranslationStandardAxis=+Y  TranslationCartesianOffset=[0 0 0]  TranslationROffset=0  TranslationROffsetUnits=m  TranslationZOffset=0  TranslationZOffsetUnits=m  TranslationThetaOffset=0  TranslationThetaOffsetUnits=deg  RotationMethod=None  RotationAngleUnits=deg  RotationStandardAxis=+Z  RotationAngle=0.0  RotationArbitraryAxis=[0 0 1]  FollAlignAxisA=+X  BaseAlignAxisA=+Y  FollAlignAxisB=+Y  BaseAlignAxisB=+Z  RotationSequenceAxes=FollowerAxes  RotationSequence=XYX  RotationSequenceAngles=[0 0 0]  RotationSequenceAnglesUnits=deg  RotationMatrix=[1 0 0; 0 1 0; 0 0 1]
  Transform FlangeR L : sm_lib/Frames and Transforms/Rigid Transform  TranslationMethod=StandardAxis  TranslationStandardOffset=(offset_l)*flfrontrear  TranslationLengthUnit=cm  TranslationStandardAxis=+X  TranslationCartesianOffset=[0 0 0]  TranslationROffset=0  TranslationROffsetUnits=m  TranslationZOffset=0  TranslationZOffsetUnits=m  TranslationThetaOffset=0  TranslationThetaOffsetUnits=deg  RotationMethod=None  RotationAngleUnits=deg  RotationStandardAxis=+Z  RotationAngle=0.0  RotationArbitraryAxis=[0 0 1]  FollAlignAxisA=+X  BaseAlignAxisA=+Y  FollAlignAxisB=+Y  BaseAlignAxisB=+Z  RotationSequenceAxes=FollowerAxes  RotationSequence=XYX  RotationSequenceAngles=[0 0 0]  RotationSequenceAnglesUnits=deg  RotationMatrix=[1 0 0; 0 1 0; 0 0 1]
  B : PMIOPort  Side=Right
  F : PMIOPort  Port=2  Side=Right
  C : PMIOPort  Port=3  Side=Left
  connections:
  Shaft R/LConn1 -- Shaft L/RConn1 -- C/RConn1
  Shaft L/LConn1 -- FlangeL/RConn1
  FlangeR/RConn1 -- Shaft R/RConn1 -- Transform FlangeR H/RConn1
  B/RConn1 -- Transform FlangeR L/LConn1
  F/RConn1 -- Transform FlangeL L/LConn1
  Transform FlangeR H/LConn1 -- Transform FlangeR L/RConn1
  Transform FlangeL H/LConn1 -- Transform FlangeL L/RConn1

== system sm_scissor_lift_lib/Brick 2 Port ==
  Solid : sm_lib/Body Elements/Brick Solid  GraphicAmbientColor=[0.15 0.15 0.15 1.0]  BasedOnType=Density  BrickDimensions=len_xyz  BrickDimensionUnits=m  CenterOfMass=[0 0 0]  CenterOfMassUnits=m  GraphicDiffuseColor=brick_clr  Density=brick_rho  DensityUnits=kg/m^3  DoExposeReferenceFrame=on  GraphicEmissiveColor=[0.0 0.0 0.0 1.0]  ExportEntireGeometry=off  SerializedFrames=<Frames/>  MarkerShape=Sphere  MarkerSize=10  GraphicType=FromGeometry  InertiaType=CalculateFromGeometry  Mass=1  MassUnits=kg  MomentsOfInertia=[1 1 1]  MomentsOfInertiaUnits=kg*m^2  GraphicOpacity=brick_opc  ProductsOfInertia=[1 1 1]  ProductsOfInertiaUnits=kg*m^2  GraphicShininess=75  GraphicSpecularColor=[0.5 0.5 0.5 1.0]  GraphicVisPropType=SimpleVisualProperties
  Transform 1 : sm_lib/Frames and Transforms/Rigid Transform  TranslationMethod=Cartesian  TranslationStandardOffset=0  TranslationLengthUnit=m  TranslationStandardAxis=+Z  TranslationCartesianOffset=port1_offset  TranslationROffset=0  TranslationROffsetUnits=m  TranslationZOffset=0  TranslationZOffsetUnits=m  TranslationThetaOffset=0  TranslationThetaOffsetUnits=deg  RotationMethod=None  RotationAngleUnits=deg  RotationStandardAxis=+Z  RotationAngle=0.0  RotationArbitraryAxis=[0 0 1]  FollAlignAxisA=+X  BaseAlignAxisA=+Y  FollAlignAxisB=+Y  BaseAlignAxisB=+Z  RotationSequenceAxes=FollowerAxes  RotationSequence=XYX  RotationSequenceAngles=[0 0 0]  RotationSequenceAnglesUnits=deg  RotationMatrix=[1 0 0; 0 1 0; 0 0 1]
  Transform 2 : sm_lib/Frames and Transforms/Rigid Transform  TranslationMethod=Cartesian  TranslationStandardOffset=0  TranslationLengthUnit=m  TranslationStandardAxis=+Z  TranslationCartesianOffset=port2_offset  TranslationROffset=0  TranslationROffsetUnits=m  TranslationZOffset=0  TranslationZOffsetUnits=m  TranslationThetaOffset=0  TranslationThetaOffsetUnits=deg  RotationMethod=None  RotationAngleUnits=deg  RotationStandardAxis=+Z  RotationAngle=0.0  RotationArbitraryAxis=[0 0 1]  FollAlignAxisA=+X  BaseAlignAxisA=+Y  FollAlignAxisB=+Y  BaseAlignAxisB=+Z  RotationSequenceAxes=FollowerAxes  RotationSequence=XYX  RotationSequenceAngles=[0 0 0]  RotationSequenceAnglesUnits=deg  RotationMatrix=[1 0 0; 0 1 0; 0 0 1]
  1X : PMIOPort  Side=Left
  X2 : PMIOPort  Port=2  Side=Right
  connections:
  X2/RConn1 -- Transform 2/RConn1
  Transform 2/LConn1 -- Transform 1/LConn1 -- Solid/RConn1
  Transform 1/RConn1 -- 1X/RConn1

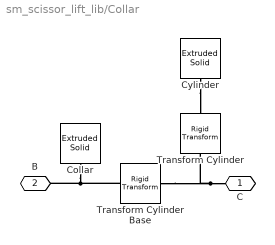
== system sm_scissor_lift_lib/Collar ==
  Collar : sm_lib/Body Elements/Extruded Solid  GraphicAmbientColor=[0.15 0.15 0.15 1.0]  BasedOnType=Density  CenterOfMass=[0 0 0]  CenterOfMassUnits=m  GraphicDiffuseColor=material_color  ExportConvexHullGeometry=off  ExtrusionCrossSection=Extr_Data_Ring(collar_radius,collar_radius*0.9,0,360)  ExtrusionCrossSectionUnits=cm  Density=material_density  DensityUnits=kg/(m^3)  DoExposeReferenceFrame=on  GraphicEmissiveColor=[0.0 0.0 0.0 1.0]  ExportEntireGeometry=off  ExtrusionLength=collar_length  ExtrusionLengthUnits=cm  ExtrusionType=General  SerializedFrames=<Frames/>  MarkerShape=Sphere  MarkerSize=10  GraphicType=FromGeometry  InertiaType=CalculateFromGeometry  Mass=1  MassUnits=kg  MomentsOfInertia=[1 1 1]  MomentsOfInertiaUnits=kg*m^2  PolygonNumSides=3  GraphicOpacity=material_opacity  PolygonOuterRadius=1  PolygonOuterRadiusUnits=m  ProductsOfInertia=[0 0 0]  ProductsOfInertiaUnits=kg*m^2  GraphicShininess=75  GraphicSpecularColor=[0.5 0.5 0.5 1.0]  GraphicVisPropType=SimpleVisualProperties
  Cylinder : sm_lib/Body Elements/Extruded Solid  GraphicAmbientColor=[0.15 0.15 0.15 1.0]  BasedOnType=Density  CenterOfMass=[0 0 0]  CenterOfMassUnits=m  GraphicDiffuseColor=material_color  ExportConvexHullGeometry=off  ExtrusionCrossSection=Extr_Data_Ring(cylinder_radius,cylinder_radius*0.9,0,360)  ExtrusionCrossSectionUnits=cm  Density=material_density  DensityUnits=kg/(m^3)  DoExposeReferenceFrame=on  GraphicEmissiveColor=[0.0 0.0 0.0 1.0]  ExportEntireGeometry=off  ExtrusionLength=cylinder_length  ExtrusionLengthUnits=cm  ExtrusionType=General  SerializedFrames=<Frames/>  MarkerShape=Sphere  MarkerSize=10  GraphicType=FromGeometry  InertiaType=CalculateFromGeometry  Mass=1  MassUnits=kg  MomentsOfInertia=[1 1 1]  MomentsOfInertiaUnits=kg*m^2  PolygonNumSides=3  GraphicOpacity=material_opacity  PolygonOuterRadius=1  PolygonOuterRadiusUnits=m  ProductsOfInertia=[0 0 0]  ProductsOfInertiaUnits=kg*m^2  GraphicShininess=75  GraphicSpecularColor=[0.5 0.5 0.5 1.0]  GraphicVisPropType=SimpleVisualProperties
  Transform Cylinder : sm_lib/Frames and Transforms/Rigid Transform  TranslationMethod=StandardAxis  TranslationStandardOffset=cylinder_length/2*cylinder_ori  TranslationLengthUnit=cm  TranslationStandardAxis=+Z  TranslationCartesianOffset=[0 0 0]  TranslationROffset=0  TranslationROffsetUnits=m  TranslationZOffset=0  TranslationZOffsetUnits=m  TranslationThetaOffset=0  TranslationThetaOffsetUnits=deg  RotationMethod=None  RotationAngleUnits=deg  RotationStandardAxis=+Y  RotationAngle=0  RotationArbitraryAxis=[0 0 1]  FollAlignAxisA=+X  BaseAlignAxisA=+Y  FollAlignAxisB=+Y  BaseAlignAxisB=+Z  RotationSequenceAxes=FollowerAxes  RotationSequence=XYX  RotationSequenceAngles=[0 0 0]  RotationSequenceAnglesUnits=deg  RotationMatrix=[1 0 0; 0 1 0; 0 0 1]
  Transform Cylinder Base : sm_lib/Frames and Transforms/Rigid Transform  TranslationMethod=None  TranslationStandardOffset=0  TranslationLengthUnit=m  TranslationStandardAxis=+Z  TranslationCartesianOffset=[0 0 0]  TranslationROffset=0  TranslationROffsetUnits=m  TranslationZOffset=0  TranslationZOffsetUnits=m  TranslationThetaOffset=0  TranslationThetaOffsetUnits=deg  RotationMethod=StandardAxis  RotationAngleUnits=deg  RotationStandardAxis=-Y  RotationAngle=90  RotationArbitraryAxis=[0 0 1]  FollAlignAxisA=+X  BaseAlignAxisA=+Y  FollAlignAxisB=+Y  BaseAlignAxisB=+Z  RotationSequenceAxes=FollowerAxes  RotationSequence=XYX  RotationSequenceAngles=[0 0 0]  RotationSequenceAnglesUnits=deg  RotationMatrix=[1 0 0; 0 1 0; 0 0 1]
  C : PMIOPort  Side=Right
  B : PMIOPort  Port=2  Side=Left
  connections:
  Transform Cylinder Base/LConn1 -- Collar/RConn1 -- B/RConn1
  Cylinder/RConn1 -- Transform Cylinder/RConn1
  C/RConn1 -- Transform Cylinder Base/RConn1 -- Transform Cylinder/LConn1

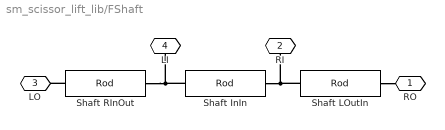
== system sm_scissor_lift_lib/FShaft ==
  Shaft InIn : $bdroot/Rod  rod_rad=shaft_radius*1e-2  rod_len=(sep_outer_outer-2*sep_outer_inner)*1e-2  rod_rho=shaft_density  rod_color=shaft_color  rod_opc=shaft_opacity  popup_zori=Local -Z  popup_markings=None  mark_radius_range=[0.5 1.01]  mark_length_range=1.005  mark_angle_range=30  mark_color=[1 1 1]
  Shaft LOutIn : $bdroot/Rod  rod_rad=shaft_radius*1e-2  rod_len=sep_outer_inner*1e-2  rod_rho=shaft_density  rod_color=shaft_color  rod_opc=shaft_opacity  popup_zori=Local -Z  popup_markings=None  mark_radius_range=[0.5 1.01]  mark_length_range=1.005  mark_angle_range=30  mark_color=[1 1 1]
  Shaft RInOut : $bdroot/Rod  rod_rad=shaft_radius*1e-2  rod_len=sep_outer_inner*1e-2  rod_rho=shaft_density  rod_color=shaft_color  rod_opc=shaft_opacity  popup_zori=Local -Z  popup_markings=None  mark_radius_range=[0.5 1.01]  mark_length_range=1.005  mark_angle_range=30  mark_color=[1 1 1]
  RO : PMIOPort  Side=Right
  RI : PMIOPort  Port=2  Side=Right
  LO : PMIOPort  Port=3  Side=Left
  LI : PMIOPort  Port=4  Side=Left
  connections:
  Shaft RInOut/RConn1 -- LO/RConn1
  Shaft LOutIn/LConn1 -- RO/RConn1
  Shaft RInOut/LConn1 -- LI/RConn1 -- Shaft InIn/RConn1
  Shaft InIn/LConn1 -- Shaft LOutIn/RConn1 -- RI/RConn1

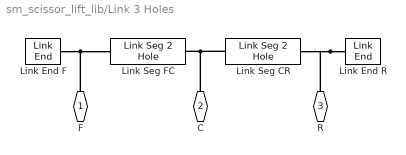
== system sm_scissor_lift_lib/Link 3 Holes ==
  Link End F : $bdroot/Link End  circ_radout=W/2*1e-2  circ_radin=r*1e-2  popup_holelr=-X  deg_1=90  deg_2=270  circ_len=T*1e-2  circ_rho=rho*1e-2  circ_color=clr  circ_opc=opc
  Link End R : $bdroot/Link End  circ_radout=W/2*1e-2  circ_radin=r*1e-2  popup_holelr=+X  deg_1=-90  deg_2=90  circ_len=T*1e-2  circ_rho=rho  circ_color=clr  circ_opc=opc
  Link Seg CR : $bdroot/Link Seg 2 Hole  link_len=L/2*1e-2  link_width=W*1e-2  link_radh=r*1e-2  link_thickness=T*1e-2  link_rho=rho  link_color=clr  link_opc=opc
  Link Seg FC : $bdroot/Link Seg 2 Hole  link_len=L/2*1e-2  link_width=W*1e-2  link_radh=r*1e-2  link_thickness=T*1e-2  link_rho=rho  link_color=clr  link_opc=opc
  F : PMIOPort  Side=Right
  C : PMIOPort  Port=2  Side=Right
  R : PMIOPort  Port=3  Side=Right
  connections:
  Link Seg FC/RConn1 -- Link Seg CR/LConn1 -- C/RConn1
  Link End F/LConn1 -- F/RConn1 -- Link Seg FC/LConn1
  Link End R/LConn1 -- Link Seg CR/RConn1 -- R/RConn1
